simulink model "PWM_multiple_fixed"  (R2023a)
settings: Solver=VariableStepAuto  StartTime=0.0  StopTime=50  MaxStep=1e-4  RelTol=1e-3
libraries: simulink x4
settings Model: Creator=Dell  LastModifiedBy=dhana
settings RTWCC: GPUComputeCapability=5.0

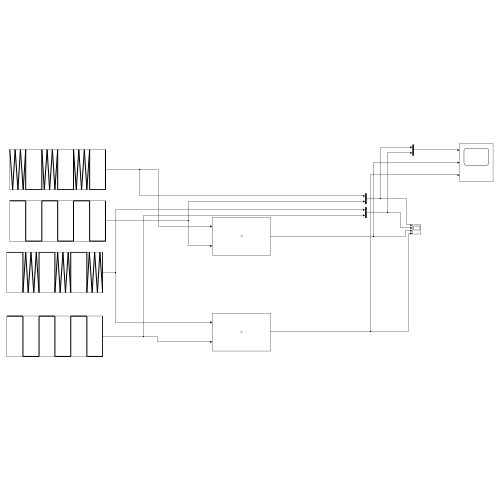
[thumbnail: Simulink's stored preview of the top-level diagram]
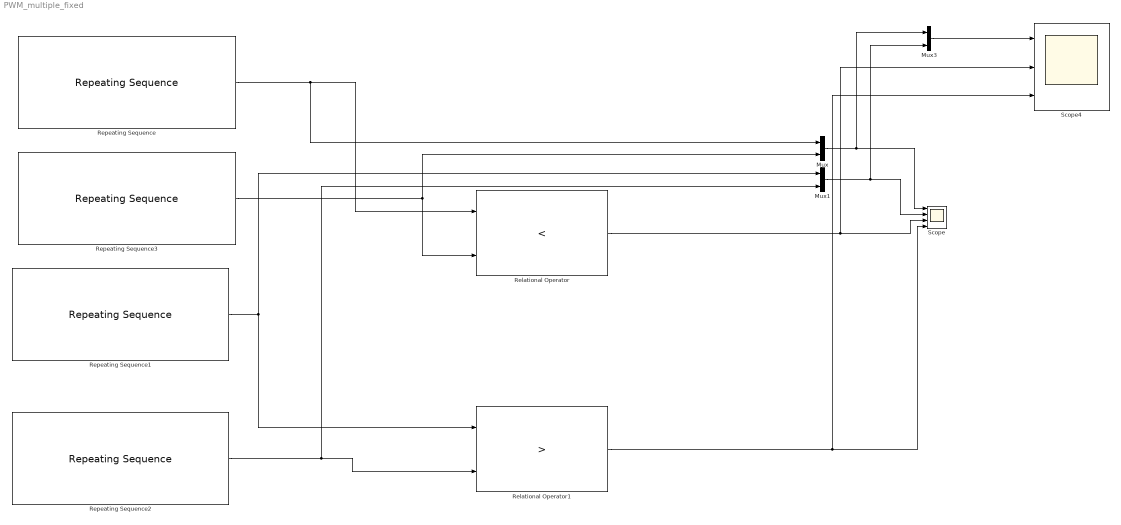
== system PWM_multiple_fixed ==
  Mux : Mux  Inputs=2
  Mux1 : Mux  Inputs=2
  Mux3 : Mux  Inputs=2
  Relational Operator : RelationalOperator  Operator=<  OutDataTypeStr=boolean  RndMeth=Simplest  InputSameDT=off
  Relational Operator1 : RelationalOperator  Operator=>  OutDataTypeStr=boolean  RndMeth=Simplest  InputSameDT=off
  Repeating Sequence : simulink/Sources/Repeating Sequence  rep_seq_t="[0 1 2 3 4 5 6 6.0001 7 8 9 10  11 12]"  rep_seq_y="[1 0 1 0 1 0 1 0 0 0 0 0  0 0 ]"
  Repeating Sequence1 : simulink/Sources/Repeating Sequence  rep_seq_t="[0 1 2 3 4 5 6 6.0001 7 8 9 10  11 12 12.0001]"  rep_seq_y="[0 0 0 0 0 0 0 -1 0 -1 0 -1  0 -1 0 ]"
  Repeating Sequence2 : simulink/Sources/Repeating Sequence  rep_seq_t=[0 6 6.0001 12 12.0001 ]  rep_seq_y="[0 0 -0.8  -0.8 0 ]"
  Repeating Sequence3 : simulink/Sources/Repeating Sequence  rep_seq_t=[0 6 6.0001 7 12 ]  rep_seq_y=[0.8 0.8 0 0 0 ]
  Scope : Scope  NumInputPorts=4
  Scope4 : Scope  NumInputPorts=3
  wires:
  Mux/1 -> Mux3/1, Scope/1
  Repeating Sequence/1 -> Mux/1, Relational Operator/1
  Repeating Sequence3/1 -> Mux/2, Relational Operator/2
  Repeating Sequence1/1 -> Relational Operator1/1, Mux1/1
  Relational Operator/1 -> Scope4/2, Scope/3
  Relational Operator1/1 -> Scope4/3, Scope/4
  Repeating Sequence2/1 -> Mux1/2, Relational Operator1/2
  Mux1/1 -> Mux3/2, Scope/2
  Mux3/1 -> Scope4/1
